simulink model "Experiment_9"  (R2021b)
settings: Solver=VariableStepAuto  StartTime=0.0  StopTime=10.0  RelTol=1e-3
settings Model: Creator=jimta  LastModifiedBy=jimta

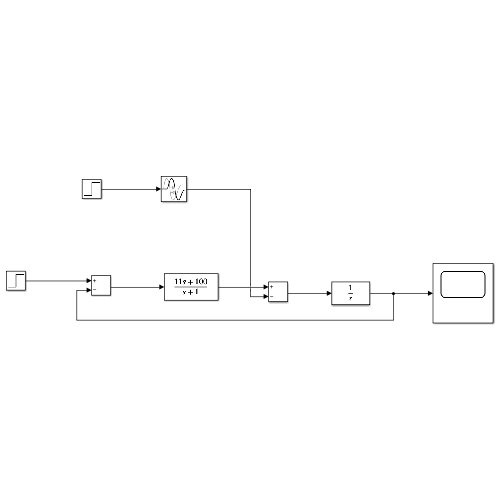
[thumbnail: Simulink's stored preview of the top-level diagram]
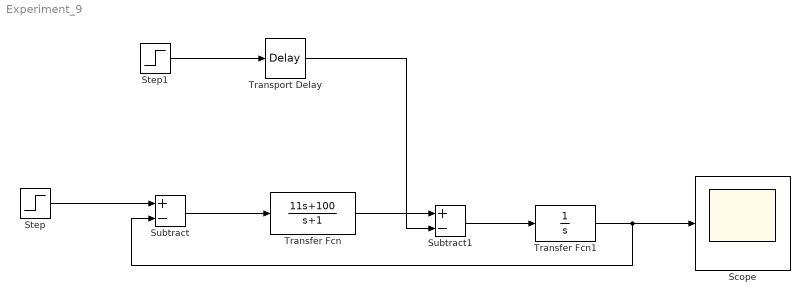
== system Experiment_9 ==
  Scope : Scope
  Step : Step  Time=0  SampleTime=0
  Step1 : Step  Time=0.3  SampleTime=0
  Subtract : Sum  Inputs=+-
  Subtract1 : Sum  Inputs=+-
  Transfer Fcn : TransferFcn  Numerator=[11 100]  Denominator=[1 1]
  Transfer Fcn1 : TransferFcn  Denominator=[1 0]
  Transport Delay : TransportDelay
  wires:
  Step1/1 -> Transport Delay/1
  Step/1 -> Subtract/1
  Subtract/1 -> Transfer Fcn/1
  Subtract1/1 -> Transfer Fcn1/1
  Transfer Fcn1/1 -> Subtract/2, Scope/1
  Transport Delay/1 -> Subtract1/2
  Transfer Fcn/1 -> Subtract1/1
